simulink model "System Modelling - Compensated - SimMechanics"  (R2015b)
settings: Solver=VariableStepAuto  StartTime=0.0  StopTime=10.0  RelTol=1e-3
libraries: mblibv1 x13, simulink x1
settings Model: Creator=acer  LastModifiedBy=acer
settings SimMechanicsCC: VisDuringSimulation=on

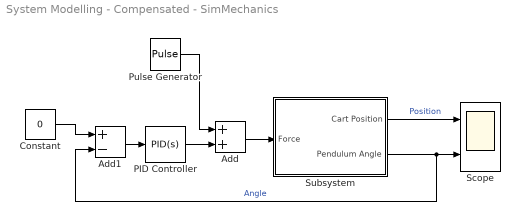
== system System Modelling - Compensated - SimMechanics ==
  Add : Sum
  Add1 : Sum  Inputs=+-
  Constant : Constant  Value=0
  PID Controller : simulink/Continuous/PID Controller  Controller=PID  TimeDomain=Continuous-time  SampleTime=-1  IntegratorMethod=Forward Euler  FilterMethod=Forward Euler  Form=Parallel  UseFilter=on  ControllerParametersSource=internal  P=13.52895  I=4.4204  D=6.332  N=100  InitialConditionSource=internal  InitialConditionForIntegrator=0  InitialConditionForFilter=0  ExternalReset=none  LimitOutput=off  UpperSaturationLimit=inf  LowerSaturationLimit=-inf  LinearizeAsGain=on  AntiWindupMode=none  Kb=1  TrackingMode=off  Kt=1  PParamMin=[]  PParamMax=[]  IParamMin=[]  IParamMax=[]  DParamMin=[]  DParamMax=[]  NParamMin=[]  NParamMax=[]  KbParamMin=[]  KbParamMax=[]  KtParamMin=[]  KtParamMax=[]  POutMin=[]  POutMax=[]  IOutMin=[]  IOutMax=[]  DOutMin=[]  DOutMax=[]  NOutMin=[]  NOutMax=[]  KbOutMin=[]  KbOutMax=[]  KtOutMin=[]  KtOutMax=[]  IntegratorOutMin=[]  IntegratorOutMax=[]  FilterOutMin=[]  FilterOutMax=[]  SumOutMin=[]  SumOutMax=[]  SumI1OutMin=[]  SumI1OutMax=[]  SumI2OutMin=[]  SumI2OutMax=[]  SumI3OutMin=[]  SumI3OutMax=[]  SumDOutMin=[]  SumDOutMax=[]  SaturationOutMin=[]  SaturationOutMax=[]  IntegratorContinuousStateAttributes=''  IntegratorStateMustResolveToSignalObject=off  IntegratorRTWStateStorageClass=Auto  FilterContinuousStateAttributes=''  FilterStateMustResolveToSignalObject=off  FilterRTWStateStorageClass=Auto  DifferentiatorICPrevScaledInput=0  DifferentiatorOutMin=[]  DifferentiatorOutMax=[]
  Pulse Generator : DiscretePulseGenerator  PulseType=Time based  Amplitude=1000  Period=10  PulseWidth=0.001
  Scope : Scope  NumInputPorts=2
  Subsystem : Subsystem
  wires:
  Subsystem/1(Cart Position) -> Scope/1  "Position"
  Subsystem/2(Pendulum Angle) -> Add1/2, Scope/2  "Angle"
  PID Controller/1 -> Add/2
  Pulse Generator/1 -> Add/1
  Add/1 -> Subsystem/1(Force)
  Add1/1 -> PID Controller/1
  Constant/1 -> Add1/1

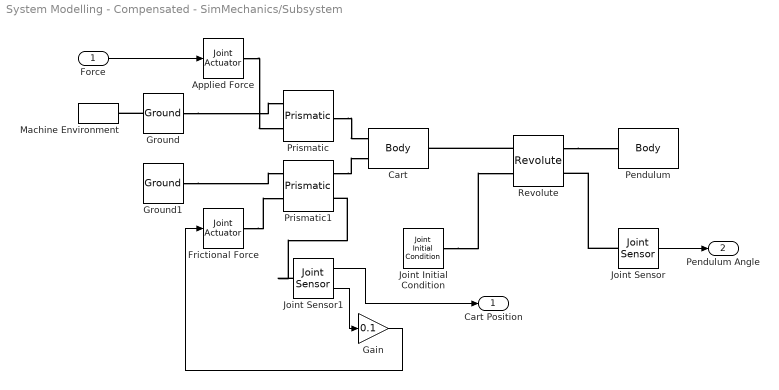
== system System Modelling - Compensated - SimMechanics/Subsystem ==
  Force : Inport
  Applied Force : mblibv1/Sensors &  Actuators/Joint Actuator  UpdateFromCAD=off  PhysicalDomain=Mechanical  PortType=blob  ActuationStyle=Force  AngleUnits=deg  ArcVelocityUnits=deg/s  ArcAccelerationUnits=deg/s^2  CoordPositionUnits=m  VelocityUnits=m/s  AccelerationUnits=m/s^2  ForceUnits=N  TorqueUnits=N-m  ActiveIO=on  Width=1  DialogClass=MechanicalActuatorBlock  Primitive=P1  ReferenceFrame=Absolute (World)
  Cart : mblibv1/Bodies/Body  LConnTagsString=CS1|CS2  RConnTagsString=CS3  UpdateFromCAD=off  DialogClass=MechanicalBodyBlock  Mass=0.5  MassUnits=kg  InertiaUnits=kg*m^2  Inertia=eye(3)  Shape=Cylinder  ShapeDims=[1 1]  ShapeUnits=m  ShapeUse=false  Density=1  DensityUnits=kg/m^3  DensityUse=false  GraphicsMode=MACHINE_DEFAULT  BodyColorSelMode=COLORPALETTE  BodyColor=[0.0705882;0.211765;0.141176]  AttachedToCS=CG  CG=Left$CG$[0 0 0]$WORLD$WORLD$m$[0 0 0]$Euler X-Y-Z$deg$WORLD$false$none  WorkingFrames=Right$CS3$[0 0.5 0]$CG$CG$m$[0 0 0]$Euler X-Y-Z$deg$WORLD$true$none#Right$CS4$[-1 0.5 0]$CG$CG$m$[0 0 0]$Euler X-Y-Z$deg$WORLD$false$none#Right$CS5$[-1 -0.5 0]$CG$CG$m$[0 0 0]$Euler X-Y-Z$deg$WORLD$false$none#Right$CS6$[1 -0.5 0]$CG$CG$m$[0 0 0]$Euler X-Y-Z$deg$WORLD$false$none#Right$CS7$[1 0.5 0]$CG$CG$m$[0 0 0]$Euler X-Y-Z$deg$WORLD$false$none#Left$CS1$[-1 0 0]$CG$CG$m$[0 0 0]$Euler X-Y-Z$deg$WORLD$true$none#Left$CS2$[0 0 0]$CG$CG$m$[0 0 0]$Euler X-Y-Z$deg$WORLD$true$none  CGPos=[0 0 0]  CGRot=[0 0 0]  CS0Pos=[]  CS0Rot=[]  CS1Pos=[-1 0 0]  CS1Rot=[0 0 0]  CS2Pos=[0 0 0]  CS2Rot=[0 0 0]  CS3Pos=[0 0.5 0]  CS3Rot=[0 0 0]  CS4Pos=[-1 0.5 0]  CS4Rot=[0 0 0]  CS5Pos=[-1 -0.5 0]  CS5Rot=[0 0 0]  CS6Pos=[1 -0.5 0]  CS6Rot=[0 0 0]  CS7Pos=[1 0.5 0]  CS7Rot=[0 0 0]  CS8Pos=[]  CS8Rot=[]  CS9Pos=[]  CS9Rot=[]  CS10Pos=[]  CS10Rot=[]  CS11Pos=[]  CS11Rot=[]  CS12Pos=[]  CS12Rot=[]  CS13Pos=[]  CS13Rot=[]  CS14Pos=[]  CS14Rot=[]  CS15Pos=[]  CS15Rot=[]  CS16Pos=[]  CS16Rot=[]  CS17Pos=[]  CS17Rot=[]  CS18Pos=[]  CS18Rot=[]  CS19Pos=[]  CS19Rot=[]  CS20Pos=[]  CS20Rot=[]
  Frictional Force : mblibv1/Sensors &  Actuators/Joint Actuator  UpdateFromCAD=off  PhysicalDomain=Mechanical  PortType=blob  ActuationStyle=Force  AngleUnits=deg  ArcVelocityUnits=deg/s  ArcAccelerationUnits=deg/s^2  CoordPositionUnits=m  VelocityUnits=m/s  AccelerationUnits=m/s^2  ForceUnits=N  TorqueUnits=N-m  ActiveIO=on  Width=1  DialogClass=MechanicalActuatorBlock  Primitive=P1  ReferenceFrame=Absolute (World)
  Gain : Gain  Gain=0.1
  Ground : mblibv1/Bodies/Ground  UpdateFromCAD=off  LeftPortType=env  RightPortType=workingframe  PhysicalDomain=Mechanical  DialogClass=GroundBlock  CoordPosition=[0 0 0]  CoordPositionUnits=m  StateVectorMgrId=0  MachineId=[1 0]  ShowEnvPort=on  ParameterChecksum=[2547200599, 2572095595, 1102623661, 3820133539]  TopologyChecksum=[3900706620, 2364327702, 1373830289, 2561305008]
  Ground1 : mblibv1/Bodies/Ground  UpdateFromCAD=off  LeftPortType=env  RightPortType=workingframe  PhysicalDomain=Mechanical  DialogClass=GroundBlock  CoordPosition=[0 0 0]  CoordPositionUnits=m  StateVectorMgrId=-1  MachineId=[0 0]  ShowEnvPort=off  ParameterChecksum=[0 0 0 0]  TopologyChecksum=[0 0 0 0]
  Joint Initial Condition : mblibv1/Sensors &  Actuators/Joint Initial Condition  UpdateFromCAD=off  LeftPortType=blob  RightPortType=blob  PhysicalDomain=mechanical  DialogClass=InitialConditionBlock  InitialConditions=P1$false$0$m$deg$0$m/s$deg/s#P2$false$0$m$deg$0$m/s$deg/s#P3$false$0$m$deg$0$m/s$deg/s#R1$true$0$m$deg$0$m/s$deg/s#R2$false$0$m$deg$0$m/s$deg/s#R3$false$0$m$deg$0$m/s$deg/s#S$false$0$m$deg$0$m/s$deg/s  P1PIC=0  P1VIC=0  P2PIC=0  P2VIC=0  P3PIC=0  P3VIC=0  R1PIC=0  R1VIC=0  R2PIC=0  R2VIC=0  R3PIC=0  R3VIC=0  SPIC=0  SVIC=0
  Joint Sensor : mblibv1/Sensors &  Actuators/Joint Sensor  UpdateFromCAD=off  PhysicalDomain=Mechanical  PortType=blob  Muxed=on  Pose=off  Angle=on  AngleUnits=rad  ArcVelocity=off  ArcVelocityUnits=deg/s  ArcAcceleration=off  ArcAccelerationUnits=deg/s^2  CoordPosition=on  CoordPositionUnits=m  Velocity=off  VelocityUnits=m/s  Acceleration=off  AccelerationUnits=m/s^2  Quaternion=on  QuaternionDT=off  QuaternionDDT=off  QuaternionUnits=off  OutputVector=[1]  ActiveIO=on  Width=1  DialogClass=MechanicalSensorBlock  Primitive=R1  Force=off  ForceUnits=N  Torque=off  TorqueUnits=N*m  ReferenceFrame=Absolute (World)  ReactionSensedSide=Base  ReactionReferenceFrame=Absolute (World)  ReactionForce=off  ReactionForceUnits=N  ReactionMoment=off  ReactionMomentUnits=N*m
  Joint Sensor1 : mblibv1/Sensors &  Actuators/Joint Sensor  UpdateFromCAD=off  PhysicalDomain=Mechanical  PortType=blob  Muxed=off  Pose=off  Angle=on  AngleUnits=deg  ArcVelocity=off  ArcVelocityUnits=deg/s  ArcAcceleration=off  ArcAccelerationUnits=deg/s^2  CoordPosition=on  CoordPositionUnits=m  Velocity=on  VelocityUnits=m/s  Acceleration=off  AccelerationUnits=m/s^2  Quaternion=on  QuaternionDT=off  QuaternionDDT=off  QuaternionUnits=off  OutputVector=[1]  ActiveIO=on  Width=2  DialogClass=MechanicalSensorBlock  Primitive=P1  Force=off  ForceUnits=N  Torque=off  TorqueUnits=N*m  ReferenceFrame=Absolute (World)  ReactionSensedSide=Base  ReactionReferenceFrame=Absolute (World)  ReactionForce=off  ReactionForceUnits=N  ReactionMoment=off  ReactionMomentUnits=N*m
  Machine Environment : mblibv1/Bodies/Machine Environment  PortType=env  PhysicalDomain=Mechanical  DialogTemplateClass=MECH.MachineEnvironment  SyncWhenCopied=off  Gravity=[0 -9.81 0]  GravityUnits=m/s^2  GravityAsSignal=off  Dimensionality=Auto-detect  AnalysisType=Forward dynamics  LinearAssemblyTolerance=1e-3  LinearAssemblyToleranceUnits=m  AngularAssemblyTolerance=1e-3  AngularAssemblyToleranceUnits=rad  ConstraintSolverType=Stabilizing  ConstraintRelTolerance=1e-4  ConstraintAbsTolerance=1e-4  UseRobustSingularityHandling=off  RedundancyAnalysisToleranceType=Automatically select tolerance  RedundancyAnalysisTolerance=1e-14  StatePerturbationType=Fixed  PerturbationSize=1e-5  VisualizeMachine=on  BodyVisualizationType=Use model default body geometries  BodyColorSelMode=Use model default  DefaultBodyColor=[1 0 0]
  Pendulum : mblibv1/Bodies/Body  LConnTagsString=CS1  UpdateFromCAD=off  DialogClass=MechanicalBodyBlock  Mass=0.2  MassUnits=kg  InertiaUnits=kg*m^2  Inertia=0.006*eye(3)  Shape=Cylinder  ShapeDims=[1 1]  ShapeUnits=m  ShapeUse=false  Density=1  DensityUnits=kg/m^3  DensityUse=false  GraphicsMode=MACHINE_DEFAULT  BodyColorSelMode=COLORPALETTE  BodyColor=[0.466667;0.67451;0.188235]  AttachedToCS=CG  CG=Left$CG$[0 0.3 0]$CS1$CS1$m$[0 0 0]$Euler X-Y-Z$deg$WORLD$false$none  WorkingFrames=Left$CS1$[0 0 0]$Adjoining$Adjoining$m$[0 0 0]$Euler X-Y-Z$deg$WORLD$true$none#Right$CS2$[0.1 0 0]$CS1$CS1$m$[0 0 0]$Euler X-Y-Z$deg$WORLD$false$none#Right$CS5$[0.1 0.6 0]$CS1$CS1$m$[0 0 0]$Euler X-Y-Z$deg$WORLD$false$none#Right$CS4$[-0.1 0.6 0]$CS1$CS1$m$[0 0 0]$Euler X-Y-Z$deg$WORLD$false$none#Right$CS3$[-0.1 0 0]$CS1$CS1$m$[0 0 0]$Euler X-Y-Z$deg$WORLD$false$none  CGPos=[0 0.3 0]  CGRot=[0 0 0]  CS0Pos=[]  CS0Rot=[]  CS1Pos=[0 0 0]  CS1Rot=[0 0 0]  CS2Pos=[0.1 0 0]  CS2Rot=[0 0 0]  CS3Pos=[-0.1 0 0]  CS3Rot=[0 0 0]  CS4Pos=[-0.1 0.6 0]  CS4Rot=[0 0 0]  CS5Pos=[0.1 0.6 0]  CS5Rot=[0 0 0]  CS6Pos=[]  CS6Rot=[]  CS7Pos=[]  CS7Rot=[]  CS8Pos=[]  CS8Rot=[]  CS9Pos=[]  CS9Rot=[]  CS10Pos=[]  CS10Rot=[]  CS11Pos=[]  CS11Rot=[]  CS12Pos=[]  CS12Rot=[]  CS13Pos=[]  CS13Rot=[]  CS14Pos=[]  CS14Rot=[]  CS15Pos=[]  CS15Rot=[]  CS16Pos=[]  CS16Rot=[]  CS17Pos=[]  CS17Rot=[]  CS18Pos=[]  CS18Rot=[]  CS19Pos=[]  CS19Rot=[]  CS20Pos=[]  CS20Rot=[]
  Prismatic : mblibv1/Joints/Prismatic  LConnTagsString=__newl0|SA1  RConnTagsString=__newr0  UpdateFromCAD=off  NumSAPorts=1  CutJoint=off  MarkAsCut=off  Primitives=prismatic  PrimitiveProps=P1$World$[1 0 0]$prismatic  DialogClass=JointBlock  P1Axis=[1 0 0]
  Prismatic1 : mblibv1/Joints/Prismatic  LConnTagsString=__newl0|SA1  RConnTagsString=__newr0|SA1  UpdateFromCAD=off  NumSAPorts=2  CutJoint=off  MarkAsCut=off  Primitives=prismatic  PrimitiveProps=P1$World$[1 0 0]$prismatic  DialogClass=JointBlock  P1Axis=[1 0 0]
  Revolute : mblibv1/Joints/Revolute  LConnTagsString=__newl0|SA1  RConnTagsString=__newr0|SA1  UpdateFromCAD=off  NumSAPorts=2  CutJoint=off  MarkAsCut=off  Primitives=prismatic  PrimitiveProps=R1$World$[0 0 1]$revolute  DialogClass=JointBlock  R1Axis=[0 0 1]
  Cart Position : Outport
  Pendulum Angle : Outport  Port=2
  wires:
  Joint Sensor1/2 -> Gain/1
  Joint Sensor/1 -> Pendulum Angle/1
  Force/1 -> Applied Force/1
  Gain/1 -> Frictional Force/1
  Joint Sensor1/1 -> Cart Position/1
  connections:
  Ground1/RConn1 -- Prismatic1/LConn1
  Applied Force/RConn1 -- Prismatic/LConn2
  Frictional Force/RConn1 -- Prismatic1/LConn2
  Ground/RConn1 -- Prismatic/LConn1
  Joint Initial Condition/RConn1 -- Revolute/LConn2
  Ground/LConn1 -- Machine Environment/RConn1
  Prismatic/RConn1 -- Cart/LConn1
  Joint Sensor/LConn1 -- Revolute/RConn2
  Revolute/LConn1 -- Cart/RConn1
  Joint Sensor1/LConn1 -- Prismatic1/RConn2
  Revolute/RConn1 -- Pendulum/LConn1
  Prismatic1/RConn1 -- Cart/LConn2
